simulink model "Pong3D"  (R2016b)
settings: Solver=ode45  StartTime=0.0  StopTime=10.0  FixedStep=0.001  MaxStep=updateFrequency  RelTol=1e-3  EnableMultiTasking=on
values from neighbouring files (symbols this model uses):
  Ball = struct(B_field1,B_value1,B_field2,B_value2,B_field3,B_value3,     B_field4,B_value4,B_field5,B_value5)    [PingPongStructs6DOF.m]
  Contact_Forces = struct(CF_field1,CF_value1,CF_field2,CF_value2,CF_field3,CF_value3)    [PingPongStructs6DOF.m]
  g = 9.81    [PingPongStructs6DOF.m]
  m = V(2)/V(1)    [AIPlayer.m]
  Net = struct(N_field1,N_value1)    [PingPongStructs6DOF.m]
  Robot1 = struct(R1_field1,R1_value1,R1_field2,R1_value2,R1_field3,R1_value3,     R1_field4,R1_value4, R1_field5,R1_value5,R1_field6,R1_value6,     R1_field7,R1_value7,R1_field8,R1_value8,R1_field9,R1_value9,R1_field10,R1_value10,     R1_field11,R1_value11,R1_field12,R1_value12)    [PingPongStructs6DOF.m]
  Robot2 = struct(R2_field1,R2_value1,R2_field2,R2_value2,R2_field3,R2_value3,     R2_field4, R2_value4, R2_field5,R2_value5,R2_field6,R2_value6,     R2_field7, R2_value7, R2_field8, R2_value8, R2_field9, R2_value9, R2_field10, R2_value10,     R2_field11, R2_value11, R2_field12, R2_value12)    [PingPongStructs6DOF.m]
  Table = struct(T_field1,T_value1,T_field2,T_value2)    [PingPongStructs6DOF.m]
undefined symbols (not defined in the file or in its folder): X, Y, Z
libraries: sm_lib x120, nesl_utility x55, fl_lib x48, Contact_Forces_Lib x4, Parts_Lib x3
(part 4 of 5)

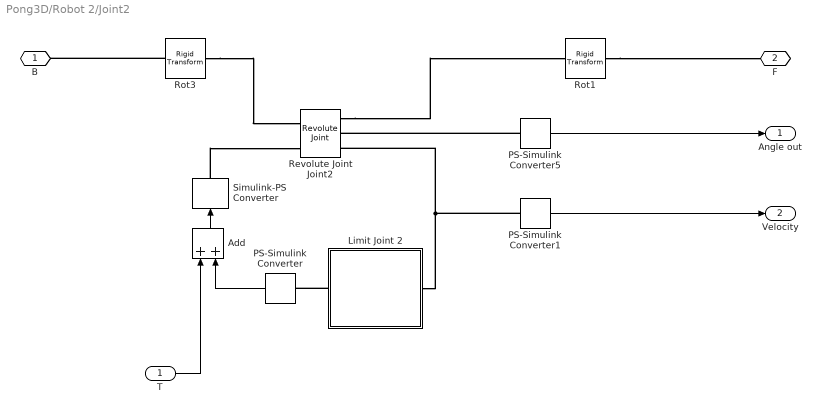
== system Pong3D/Robot 2/Joint2 ==
  T : Inport
  Add : Sum
  Limit Joint 2 : Subsystem
  PS-Simulink Converter : nesl_utility/PS-Simulink Converter  PhysicalDomain=network_engine_domain  SubClassName=ps_output  LeftPortType=input  RightPortType=output  PseudoPeriodic=off  Frequencies=[]  Unit=1  AffineConversion=off
  PS-Simulink Converter1 : nesl_utility/PS-Simulink Converter  PhysicalDomain=network_engine_domain  SubClassName=ps_output  LeftPortType=input  RightPortType=output  PseudoPeriodic=off  Frequencies=[]  Unit=1  AffineConversion=off
  PS-Simulink Converter5 : nesl_utility/PS-Simulink Converter  PhysicalDomain=network_engine_domain  SubClassName=ps_output  LeftPortType=input  RightPortType=output  PseudoPeriodic=off  Frequencies=[]  Unit=1  AffineConversion=off
  Revolute Joint Joint2 : sm_lib/Joints/Revolute Joint  SenseConstraintForce=off  SenseConstraintForceX=off  SenseConstraintForceY=off  SenseConstraintForceZ=off  SenseConstraintTorque=off  SenseConstraintTorqueX=off  SenseConstraintTorqueY=off  SenseConstraintTorqueZ=off  SenseTotalForce=off  SenseTotalForceX=off  SenseTotalForceY=off  SenseTotalForceZ=off  SenseTotalTorque=off  SenseTotalTorqueX=off  SenseTotalTorqueY=off  SenseTotalTorqueZ=off  CompositeWrenchDir=FollowerOnBase  CompositeWrenchFrame=BaseFrame  EquilibriumPosition=0  EquilibriumPositionUnits=deg  SpringStiffness=0  SpringStiffnessUnits=N*m/deg  DampingCoefficient=0  DampingCoefficientUnits=N*m/(deg/s)  TorqueActuationMode=InputTorque  MotionActuationMode=ComputedMotion  SensePosition=on  SenseVelocity=on  SenseAcceleration=off  SenseTorqueForce=off  PositionTargetSpecify=on  PositionTargetPriority=High  PositionTargetValue=Robot2.Joint.Initial_Angle(2)  PositionTargetValueUnits=deg  VelocityTargetSpecify=off  VelocityTargetPriority=High  VelocityTargetValue=0  VelocityTargetValueUnits=deg/s
  Rot1 : sm_lib/Frames and Transforms/Rigid Transform  TranslationMethod=None  TranslationStandardOffset=0  TranslationLengthUnit=m  TranslationStandardAxis=+Z  TranslationCartesianOffset=[0 0 0]  TranslationROffset=0  TranslationROffsetUnits=m  TranslationZOffset=0  TranslationZOffsetUnits=m  TranslationThetaOffset=0  TranslationThetaOffsetUnits=deg  RotationMethod=StandardAxis  RotationAngleUnits=deg  RotationStandardAxis=-X  RotationAngle=90  RotationArbitraryAxis=[0 0 1]  FollAlignAxisA=+X  BaseAlignAxisA=+Y  FollAlignAxisB=+Y  BaseAlignAxisB=+Z  RotationSequenceAxes=FollowerAxes  RotationSequence=XYX  RotationSequenceAngles=[0 0 0]  RotationSequenceAnglesUnits=deg  RotationMatrix=[1 0 0; 0 1 0; 0 0 1]
      settings: AttributesFormatString=|
      | %<RotationAngle> %<RotationAngleUnits>
      | about %<RotationStandardAxis>
  Rot3 : sm_lib/Frames and Transforms/Rigid Transform  TranslationMethod=None  TranslationStandardOffset=0  TranslationLengthUnit=m  TranslationStandardAxis=+Z  TranslationCartesianOffset=[0 0 0]  TranslationROffset=0  TranslationROffsetUnits=m  TranslationZOffset=0  TranslationZOffsetUnits=m  TranslationThetaOffset=0  TranslationThetaOffsetUnits=deg  RotationMethod=StandardAxis  RotationAngleUnits=deg  RotationStandardAxis=+X  RotationAngle=90  RotationArbitraryAxis=[0 0 1]  FollAlignAxisA=+X  BaseAlignAxisA=+Y  FollAlignAxisB=+Y  BaseAlignAxisB=+Z  RotationSequenceAxes=FollowerAxes  RotationSequence=XYX  RotationSequenceAngles=[0 0 0]  RotationSequenceAnglesUnits=deg  RotationMatrix=[1 0 0; 0 1 0; 0 0 1]
      settings: AttributesFormatString=|
      | %<RotationAngle> %<RotationAngleUnits>
      | about %<RotationStandardAxis>
  Simulink-PS Converter : nesl_utility/Simulink-PS Converter  PhysicalDomain=network_engine_domain  SubClassName=ps_input  LeftPortType=input  RightPortType=output  PseudoPeriodic=off  Frequencies=[]  NoiseDistribution=none  NoiseParameters=[]  Unit=1  AffineConversion=off  InputFiltering=off  SimscapeFilterOrder=1  InputFilterTimeConstant=0.001  UdotUserProvided=1
  B : PMIOPort  Port=1  Side=Left
  F : PMIOPort  Port=2  Side=Right
  Angle out : Outport
  Velocity : Outport  Port=2
  wires:
  Add/1 -> Simulink-PS Converter/1
  T/1 -> Add/1
  PS-Simulink Converter/1 -> Add/2
  PS-Simulink Converter5/1 -> Angle out/1
  PS-Simulink Converter1/1 -> Velocity/1
  connections:
  Rot3/LConn1 -- B/RConn1
  Limit Joint 2/RConn1 -- PS-Simulink Converter/LConn1
  Simulink-PS Converter/RConn1 -- Revolute Joint Joint2/LConn2
  Revolute Joint Joint2/RConn1 -- Rot1/LConn1
  Rot3/RConn1 -- Revolute Joint Joint2/LConn1
  Limit Joint 2/LConn1 -- PS-Simulink Converter1/LConn1 -- Revolute Joint Joint2/RConn3
  PS-Simulink Converter5/LConn1 -- Revolute Joint Joint2/RConn2
  Rot1/RConn1 -- F/RConn1

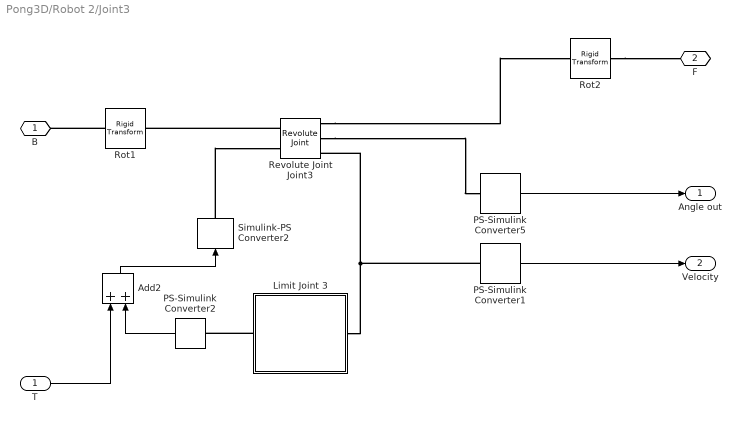
== system Pong3D/Robot 2/Joint3 ==
  T : Inport
  Add2 : Sum
  Limit Joint 3 : Subsystem
  PS-Simulink Converter1 : nesl_utility/PS-Simulink Converter  PhysicalDomain=network_engine_domain  SubClassName=ps_output  LeftPortType=input  RightPortType=output  PseudoPeriodic=off  Frequencies=[]  Unit=1  AffineConversion=off
  PS-Simulink Converter2 : nesl_utility/PS-Simulink Converter  PhysicalDomain=network_engine_domain  SubClassName=ps_output  LeftPortType=input  RightPortType=output  PseudoPeriodic=off  Frequencies=[]  Unit=1  AffineConversion=off
  PS-Simulink Converter5 : nesl_utility/PS-Simulink Converter  PhysicalDomain=network_engine_domain  SubClassName=ps_output  LeftPortType=input  RightPortType=output  PseudoPeriodic=off  Frequencies=[]  Unit=1  AffineConversion=off
  Revolute Joint Joint3 : sm_lib/Joints/Revolute Joint  SenseConstraintForce=off  SenseConstraintForceX=off  SenseConstraintForceY=off  SenseConstraintForceZ=off  SenseConstraintTorque=off  SenseConstraintTorqueX=off  SenseConstraintTorqueY=off  SenseConstraintTorqueZ=off  SenseTotalForce=off  SenseTotalForceX=off  SenseTotalForceY=off  SenseTotalForceZ=off  SenseTotalTorque=off  SenseTotalTorqueX=off  SenseTotalTorqueY=off  SenseTotalTorqueZ=off  CompositeWrenchDir=FollowerOnBase  CompositeWrenchFrame=BaseFrame  EquilibriumPosition=0  EquilibriumPositionUnits=deg  SpringStiffness=0  SpringStiffnessUnits=N*m/deg  DampingCoefficient=0  DampingCoefficientUnits=N*m/(deg/s)  TorqueActuationMode=InputTorque  MotionActuationMode=ComputedMotion  SensePosition=on  SenseVelocity=on  SenseAcceleration=off  SenseTorqueForce=off  PositionTargetSpecify=on  PositionTargetPriority=High  PositionTargetValue=Robot2.Joint.Initial_Angle(3)  PositionTargetValueUnits=deg  VelocityTargetSpecify=off  VelocityTargetPriority=High  VelocityTargetValue=0  VelocityTargetValueUnits=deg/s
  Rot1 : sm_lib/Frames and Transforms/Rigid Transform  TranslationMethod=None  TranslationStandardOffset=0  TranslationLengthUnit=m  TranslationStandardAxis=+Z  TranslationCartesianOffset=[0 0 0]  TranslationROffset=0  TranslationROffsetUnits=m  TranslationZOffset=0  TranslationZOffsetUnits=m  TranslationThetaOffset=0  TranslationThetaOffsetUnits=deg  RotationMethod=StandardAxis  RotationAngleUnits=deg  RotationStandardAxis=+X  RotationAngle=90  RotationArbitraryAxis=[0 0 1]  FollAlignAxisA=+X  BaseAlignAxisA=+Y  FollAlignAxisB=+Y  BaseAlignAxisB=+Z  RotationSequenceAxes=FollowerAxes  RotationSequence=XYX  RotationSequenceAngles=[0 0 0]  RotationSequenceAnglesUnits=deg  RotationMatrix=[1 0 0; 0 1 0; 0 0 1]
      settings: AttributesFormatString=|
      | %<RotationAngle> %<RotationAngleUnits>
      | about %<RotationStandardAxis>
  Rot2 : sm_lib/Frames and Transforms/Rigid Transform  TranslationMethod=None  TranslationStandardOffset=0  TranslationLengthUnit=m  TranslationStandardAxis=+Z  TranslationCartesianOffset=[0 0 0]  TranslationROffset=0  TranslationROffsetUnits=m  TranslationZOffset=0  TranslationZOffsetUnits=m  TranslationThetaOffset=0  TranslationThetaOffsetUnits=deg  RotationMethod=StandardAxis  RotationAngleUnits=deg  RotationStandardAxis=-X  RotationAngle=90  RotationArbitraryAxis=[0 0 1]  FollAlignAxisA=+X  BaseAlignAxisA=+Y  FollAlignAxisB=+Y  BaseAlignAxisB=+Z  RotationSequenceAxes=FollowerAxes  RotationSequence=XYX  RotationSequenceAngles=[0 0 0]  RotationSequenceAnglesUnits=deg  RotationMatrix=[1 0 0; 0 1 0; 0 0 1]
      settings: AttributesFormatString=|
      | %<RotationAngle> %<RotationAngleUnits>
      | about %<RotationStandardAxis>
  Simulink-PS Converter2 : nesl_utility/Simulink-PS Converter  PhysicalDomain=network_engine_domain  SubClassName=ps_input  LeftPortType=input  RightPortType=output  PseudoPeriodic=off  Frequencies=[]  NoiseDistribution=none  NoiseParameters=[]  Unit=1  AffineConversion=off  InputFiltering=off  SimscapeFilterOrder=1  InputFilterTimeConstant=0.001  UdotUserProvided=1
  B : PMIOPort  Port=1  Side=Left
  F : PMIOPort  Port=2  Side=Right
  Angle out : Outport
  Velocity : Outport  Port=2
  wires:
  PS-Simulink Converter2/1 -> Add2/2
  Add2/1 -> Simulink-PS Converter2/1
  T/1 -> Add2/1
  PS-Simulink Converter5/1 -> Angle out/1
  PS-Simulink Converter1/1 -> Velocity/1
  connections:
  Limit Joint 3/LConn1 -- PS-Simulink Converter1/LConn1 -- Revolute Joint Joint3/RConn3
  Revolute Joint Joint3/RConn2 -- PS-Simulink Converter5/LConn1
  Simulink-PS Converter2/RConn1 -- Revolute Joint Joint3/LConn2
  Limit Joint 3/RConn1 -- PS-Simulink Converter2/LConn1
  Rot1/LConn1 -- B/RConn1
  Revolute Joint Joint3/RConn1 -- Rot2/LConn1
  Revolute Joint Joint3/LConn1 -- Rot1/RConn1
  Rot2/RConn1 -- F/RConn1

== system Pong3D/Robot 2/Joint4 ==
  Ty : Inport
  Add3 : Sum
  Limit Joint 4 Y : Subsystem
  PS-Simulink Converter1 : nesl_utility/PS-Simulink Converter  PhysicalDomain=network_engine_domain  SubClassName=ps_output  LeftPortType=input  RightPortType=output  PseudoPeriodic=off  Frequencies=[]  Unit=1  AffineConversion=off
  PS-Simulink Converter2 : nesl_utility/PS-Simulink Converter  PhysicalDomain=network_engine_domain  SubClassName=ps_output  LeftPortType=input  RightPortType=output  PseudoPeriodic=off  Frequencies=[]  Unit=1  AffineConversion=off
  PS-Simulink Converter3 : nesl_utility/PS-Simulink Converter  PhysicalDomain=network_engine_domain  SubClassName=ps_output  LeftPortType=input  RightPortType=output  PseudoPeriodic=off  Frequencies=[]  Unit=1  AffineConversion=off
  Revolute Joint : sm_lib/Joints/Revolute Joint  SenseConstraintForce=off  SenseConstraintForceX=off  SenseConstraintForceY=off  SenseConstraintForceZ=off  SenseConstraintTorque=off  SenseConstraintTorqueX=off  SenseConstraintTorqueY=off  SenseConstraintTorqueZ=off  SenseTotalForce=off  SenseTotalForceX=off  SenseTotalForceY=off  SenseTotalForceZ=off  SenseTotalTorque=off  SenseTotalTorqueX=off  SenseTotalTorqueY=off  SenseTotalTorqueZ=off  CompositeWrenchDir=FollowerOnBase  CompositeWrenchFrame=BaseFrame  EquilibriumPosition=0  EquilibriumPositionUnits=deg  SpringStiffness=0  SpringStiffnessUnits=N*m/deg  DampingCoefficient=0  DampingCoefficientUnits=N*m/(deg/s)  TorqueActuationMode=InputTorque  MotionActuationMode=ComputedMotion  SensePosition=on  SenseVelocity=on  SenseAcceleration=off  SenseTorqueForce=off  PositionTargetSpecify=on  PositionTargetPriority=High  PositionTargetValue=Robot2.Joint.Initial_Angle(4)  PositionTargetValueUnits=deg  VelocityTargetSpecify=off  VelocityTargetPriority=High  VelocityTargetValue=0  VelocityTargetValueUnits=deg/s
  Rot1 : sm_lib/Frames and Transforms/Rigid Transform  TranslationMethod=None  TranslationStandardOffset=0  TranslationLengthUnit=m  TranslationStandardAxis=+Z  TranslationCartesianOffset=[0 0 0]  TranslationROffset=0  TranslationROffsetUnits=m  TranslationZOffset=0  TranslationZOffsetUnits=m  TranslationThetaOffset=0  TranslationThetaOffsetUnits=deg  RotationMethod=StandardAxis  RotationAngleUnits=deg  RotationStandardAxis=+X  RotationAngle=180  RotationArbitraryAxis=[0 0 1]  FollAlignAxisA=+X  BaseAlignAxisA=+Y  FollAlignAxisB=+Y  BaseAlignAxisB=+Z  RotationSequenceAxes=FollowerAxes  RotationSequence=XYX  RotationSequenceAngles=[0 0 0]  RotationSequenceAnglesUnits=deg  RotationMatrix=[1 0 0; 0 1 0; 0 0 1]
      settings: AttributesFormatString=|
      | %<RotationAngle> %<RotationAngleUnits>
      | about %<RotationStandardAxis>
  Rot2 : sm_lib/Frames and Transforms/Rigid Transform  TranslationMethod=None  TranslationStandardOffset=0  TranslationLengthUnit=m  TranslationStandardAxis=+Z  TranslationCartesianOffset=[0 0 0]  TranslationROffset=0  TranslationROffsetUnits=m  TranslationZOffset=0  TranslationZOffsetUnits=m  TranslationThetaOffset=0  TranslationThetaOffsetUnits=deg  RotationMethod=StandardAxis  RotationAngleUnits=deg  RotationStandardAxis=-X  RotationAngle=180  RotationArbitraryAxis=[0 0 1]  FollAlignAxisA=+X  BaseAlignAxisA=+Y  FollAlignAxisB=+Y  BaseAlignAxisB=+Z  RotationSequenceAxes=FollowerAxes  RotationSequence=XYX  RotationSequenceAngles=[0 0 0]  RotationSequenceAnglesUnits=deg  RotationMatrix=[1 0 0; 0 1 0; 0 0 1]
      settings: AttributesFormatString=|
      | %<RotationAngle> %<RotationAngleUnits>
      | about %<RotationStandardAxis>
  Simulink-PS Converter3 : nesl_utility/Simulink-PS Converter  PhysicalDomain=network_engine_domain  SubClassName=ps_input  LeftPortType=input  RightPortType=output  PseudoPeriodic=off  Frequencies=[]  NoiseDistribution=none  NoiseParameters=[]  Unit=1  AffineConversion=off  InputFiltering=off  SimscapeFilterOrder=1  InputFilterTimeConstant=0.001  UdotUserProvided=1
  B : PMIOPort  Port=1  Side=Left
  F : PMIOPort  Port=2  Side=Right
  Angle Y out : Outport
  Velocity : Outport  Port=2
  wires:
  Add3/1 -> Simulink-PS Converter3/1
  PS-Simulink Converter3/1 -> Add3/2
  PS-Simulink Converter1/1 -> Angle Y out/1
  Ty/1 -> Add3/1
  PS-Simulink Converter2/1 -> Velocity/1
  connections:
  Rot2/RConn1 -- F/RConn1
  Limit Joint 4 Y/RConn1 -- PS-Simulink Converter3/LConn1
  Rot1/RConn1 -- Revolute Joint/LConn1
  PS-Simulink Converter1/LConn1 -- Revolute Joint/RConn2
  Limit Joint 4 Y/LConn1 -- Revolute Joint/RConn3 -- PS-Simulink Converter2/LConn1
  Simulink-PS Converter3/RConn1 -- Revolute Joint/LConn2
  B/RConn1 -- Rot1/LConn1
  Revolute Joint/RConn1 -- Rot2/LConn1

== system Pong3D/Robot 2/Joint5 ==
  Ty : Inport
  Add3 : Sum
  Limit Joint 4 Y : Subsystem
  PS-Simulink Converter1 : nesl_utility/PS-Simulink Converter  PhysicalDomain=network_engine_domain  SubClassName=ps_output  LeftPortType=input  RightPortType=output  PseudoPeriodic=off  Frequencies=[]  Unit=1  AffineConversion=off
  PS-Simulink Converter2 : nesl_utility/PS-Simulink Converter  PhysicalDomain=network_engine_domain  SubClassName=ps_output  LeftPortType=input  RightPortType=output  PseudoPeriodic=off  Frequencies=[]  Unit=1  AffineConversion=off
  PS-Simulink Converter3 : nesl_utility/PS-Simulink Converter  PhysicalDomain=network_engine_domain  SubClassName=ps_output  LeftPortType=input  RightPortType=output  PseudoPeriodic=off  Frequencies=[]  Unit=1  AffineConversion=off
  Revolute Joint : sm_lib/Joints/Revolute Joint  SenseConstraintForce=off  SenseConstraintForceX=off  SenseConstraintForceY=off  SenseConstraintForceZ=off  SenseConstraintTorque=off  SenseConstraintTorqueX=off  SenseConstraintTorqueY=off  SenseConstraintTorqueZ=off  SenseTotalForce=off  SenseTotalForceX=off  SenseTotalForceY=off  SenseTotalForceZ=off  SenseTotalTorque=off  SenseTotalTorqueX=off  SenseTotalTorqueY=off  SenseTotalTorqueZ=off  CompositeWrenchDir=FollowerOnBase  CompositeWrenchFrame=BaseFrame  EquilibriumPosition=0  EquilibriumPositionUnits=deg  SpringStiffness=0  SpringStiffnessUnits=N*m/deg  DampingCoefficient=0  DampingCoefficientUnits=N*m/(deg/s)  TorqueActuationMode=InputTorque  MotionActuationMode=ComputedMotion  SensePosition=on  SenseVelocity=on  SenseAcceleration=off  SenseTorqueForce=off  PositionTargetSpecify=on  PositionTargetPriority=High  PositionTargetValue=Robot2.Joint.Initial_Angle(5)  PositionTargetValueUnits=deg  VelocityTargetSpecify=off  VelocityTargetPriority=High  VelocityTargetValue=0  VelocityTargetValueUnits=deg/s
  Rot1 : sm_lib/Frames and Transforms/Rigid Transform  TranslationMethod=None  TranslationStandardOffset=0  TranslationLengthUnit=m  TranslationStandardAxis=+Z  TranslationCartesianOffset=[0 0 0]  TranslationROffset=0  TranslationROffsetUnits=m  TranslationZOffset=0  TranslationZOffsetUnits=m  TranslationThetaOffset=0  TranslationThetaOffsetUnits=deg  RotationMethod=StandardAxis  RotationAngleUnits=deg  RotationStandardAxis=-X  RotationAngle=90  RotationArbitraryAxis=[0 0 1]  FollAlignAxisA=+X  BaseAlignAxisA=+Y  FollAlignAxisB=+Y  BaseAlignAxisB=+Z  RotationSequenceAxes=FollowerAxes  RotationSequence=XYX  RotationSequenceAngles=[0 0 0]  RotationSequenceAnglesUnits=deg  RotationMatrix=[1 0 0; 0 1 0; 0 0 1]
      settings: AttributesFormatString=|
      | %<RotationAngle> %<RotationAngleUnits>
      | about %<RotationStandardAxis>
  Rot3 : sm_lib/Frames and Transforms/Rigid Transform  TranslationMethod=None  TranslationStandardOffset=0  TranslationLengthUnit=m  TranslationStandardAxis=+Z  TranslationCartesianOffset=[0 0 0]  TranslationROffset=0  TranslationROffsetUnits=m  TranslationZOffset=0  TranslationZOffsetUnits=m  TranslationThetaOffset=0  TranslationThetaOffsetUnits=deg  RotationMethod=StandardAxis  RotationAngleUnits=deg  RotationStandardAxis=+X  RotationAngle=90  RotationArbitraryAxis=[0 0 1]  FollAlignAxisA=+X  BaseAlignAxisA=+Y  FollAlignAxisB=+Y  BaseAlignAxisB=+Z  RotationSequenceAxes=FollowerAxes  RotationSequence=XYX  RotationSequenceAngles=[0 0 0]  RotationSequenceAnglesUnits=deg  RotationMatrix=[1 0 0; 0 1 0; 0 0 1]
      settings: AttributesFormatString=|
      | %<RotationAngle> %<RotationAngleUnits>
      | about %<RotationStandardAxis>
  Simulink-PS Converter3 : nesl_utility/Simulink-PS Converter  PhysicalDomain=network_engine_domain  SubClassName=ps_input  LeftPortType=input  RightPortType=output  PseudoPeriodic=off  Frequencies=[]  NoiseDistribution=none  NoiseParameters=[]  Unit=1  AffineConversion=off  InputFiltering=off  SimscapeFilterOrder=1  InputFilterTimeConstant=0.001  UdotUserProvided=1
  B : PMIOPort  Port=1  Side=Left
  F : PMIOPort  Port=2  Side=Right
  Angle Y out : Outport
  Velocity : Outport  Port=2
  wires:
  Ty/1 -> Add3/1
  PS-Simulink Converter1/1 -> Angle Y out/1
  PS-Simulink Converter3/1 -> Add3/2
  Add3/1 -> Simulink-PS Converter3/1
  PS-Simulink Converter2/1 -> Velocity/1
  connections:
  Simulink-PS Converter3/RConn1 -- Revolute Joint/LConn2
  Limit Joint 4 Y/LConn1 -- PS-Simulink Converter2/LConn1 -- Revolute Joint/RConn3
  PS-Simulink Converter1/LConn1 -- Revolute Joint/RConn2
  Limit Joint 4 Y/RConn1 -- PS-Simulink Converter3/LConn1
  Revolute Joint/RConn1 -- Rot1/LConn1
  B/RConn1 -- Rot3/LConn1
  Rot3/RConn1 -- Revolute Joint/LConn1
  Rot1/RConn1 -- F/RConn1

== system Pong3D/Robot 2/Joint6 ==
  Ty : Inport
  Add3 : Sum
  Limit Joint 4 Y : Subsystem
  PS-Simulink Converter1 : nesl_utility/PS-Simulink Converter  PhysicalDomain=network_engine_domain  SubClassName=ps_output  LeftPortType=input  RightPortType=output  PseudoPeriodic=off  Frequencies=[]  Unit=1  AffineConversion=off
  PS-Simulink Converter2 : nesl_utility/PS-Simulink Converter  PhysicalDomain=network_engine_domain  SubClassName=ps_output  LeftPortType=input  RightPortType=output  PseudoPeriodic=off  Frequencies=[]  Unit=1  AffineConversion=off
  PS-Simulink Converter3 : nesl_utility/PS-Simulink Converter  PhysicalDomain=network_engine_domain  SubClassName=ps_output  LeftPortType=input  RightPortType=output  PseudoPeriodic=off  Frequencies=[]  Unit=1  AffineConversion=off
  Revolute Joint : sm_lib/Joints/Revolute Joint  SenseConstraintForce=off  SenseConstraintForceX=off  SenseConstraintForceY=off  SenseConstraintForceZ=off  SenseConstraintTorque=off  SenseConstraintTorqueX=off  SenseConstraintTorqueY=off  SenseConstraintTorqueZ=off  SenseTotalForce=off  SenseTotalForceX=off  SenseTotalForceY=off  SenseTotalForceZ=off  SenseTotalTorque=off  SenseTotalTorqueX=off  SenseTotalTorqueY=off  SenseTotalTorqueZ=off  CompositeWrenchDir=FollowerOnBase  CompositeWrenchFrame=BaseFrame  EquilibriumPosition=0  EquilibriumPositionUnits=deg  SpringStiffness=0  SpringStiffnessUnits=N*m/deg  DampingCoefficient=0  DampingCoefficientUnits=N*m/(deg/s)  TorqueActuationMode=InputTorque  MotionActuationMode=ComputedMotion  SensePosition=on  SenseVelocity=on  SenseAcceleration=off  SenseTorqueForce=off  PositionTargetSpecify=on  PositionTargetPriority=High  PositionTargetValue=Robot2.Joint.Initial_Angle(6)  PositionTargetValueUnits=deg  VelocityTargetSpecify=off  VelocityTargetPriority=High  VelocityTargetValue=0  VelocityTargetValueUnits=deg/s
  Rot1 : sm_lib/Frames and Transforms/Rigid Transform  TranslationMethod=None  TranslationStandardOffset=0  TranslationLengthUnit=m  TranslationStandardAxis=+Z  TranslationCartesianOffset=[0 0 0]  TranslationROffset=0  TranslationROffsetUnits=m  TranslationZOffset=0  TranslationZOffsetUnits=m  TranslationThetaOffset=0  TranslationThetaOffsetUnits=deg  RotationMethod=StandardAxis  RotationAngleUnits=deg  RotationStandardAxis=+X  RotationAngle=180  RotationArbitraryAxis=[0 0 1]  FollAlignAxisA=+X  BaseAlignAxisA=+Y  FollAlignAxisB=+Y  BaseAlignAxisB=+Z  RotationSequenceAxes=FollowerAxes  RotationSequence=XYX  RotationSequenceAngles=[0 0 0]  RotationSequenceAnglesUnits=deg  RotationMatrix=[1 0 0; 0 1 0; 0 0 1]
      settings: AttributesFormatString=|
      | %<RotationAngle> %<RotationAngleUnits>
      | about %<RotationStandardAxis>
  Rot2 : sm_lib/Frames and Transforms/Rigid Transform  TranslationMethod=None  TranslationStandardOffset=0  TranslationLengthUnit=m  TranslationStandardAxis=+Z  TranslationCartesianOffset=[0 0 0]  TranslationROffset=0  TranslationROffsetUnits=m  TranslationZOffset=0  TranslationZOffsetUnits=m  TranslationThetaOffset=0  TranslationThetaOffsetUnits=deg  RotationMethod=StandardAxis  RotationAngleUnits=deg  RotationStandardAxis=-X  RotationAngle=180  RotationArbitraryAxis=[0 0 1]  FollAlignAxisA=+X  BaseAlignAxisA=+Y  FollAlignAxisB=+Y  BaseAlignAxisB=+Z  RotationSequenceAxes=FollowerAxes  RotationSequence=XYX  RotationSequenceAngles=[0 0 0]  RotationSequenceAnglesUnits=deg  RotationMatrix=[1 0 0; 0 1 0; 0 0 1]
      settings: AttributesFormatString=|
      | %<RotationAngle> %<RotationAngleUnits>
      | about %<RotationStandardAxis>
  Simulink-PS Converter3 : nesl_utility/Simulink-PS Converter  PhysicalDomain=network_engine_domain  SubClassName=ps_input  LeftPortType=input  RightPortType=output  PseudoPeriodic=off  Frequencies=[]  NoiseDistribution=none  NoiseParameters=[]  Unit=1  AffineConversion=off  InputFiltering=off  SimscapeFilterOrder=1  InputFilterTimeConstant=0.001  UdotUserProvided=1
  B : PMIOPort  Port=1  Side=Left
  F : PMIOPort  Port=2  Side=Right
  Angle Y out : Outport
  Velocity : Outport  Port=2
  wires:
  Ty/1 -> Add3/1
  PS-Simulink Converter1/1 -> Angle Y out/1
  PS-Simulink Converter3/1 -> Add3/2
  Add3/1 -> Simulink-PS Converter3/1
  PS-Simulink Converter2/1 -> Velocity/1
  connections:
  Simulink-PS Converter3/RConn1 -- Revolute Joint/LConn2
  Limit Joint 4 Y/LConn1 -- PS-Simulink Converter2/LConn1 -- Revolute Joint/RConn3
  PS-Simulink Converter1/LConn1 -- Revolute Joint/RConn2
  Limit Joint 4 Y/RConn1 -- PS-Simulink Converter3/LConn1
  B/RConn1 -- Rot1/LConn1
  Rot2/RConn1 -- F/RConn1
  Rot1/RConn1 -- Revolute Joint/LConn1
  Revolute Joint/RConn1 -- Rot2/LConn1

== system Pong3D/Robot 2/Paddle1 ==
  Paddle1 : Parts_Lib/Cylinder  Tag=CustomStyle  cyl_radius=Robot2.Paddle(1)  cyl_length=Robot2.Paddle(2)  cyl_density=Robot2.Paddle(3)  cyl_color=blue  cyl_opacity=1  mark_radius=[0.75 0.5]  mark_angle=60  mark_color=purple  mark_opacity=1
  Rot1 : sm_lib/Frames and Transforms/Rigid Transform  TranslationMethod=None  TranslationStandardOffset=0  TranslationLengthUnit=m  TranslationStandardAxis=+Z  TranslationCartesianOffset=[0 0 0]  TranslationROffset=0  TranslationROffsetUnits=m  TranslationZOffset=0  TranslationZOffsetUnits=m  TranslationThetaOffset=0  TranslationThetaOffsetUnits=deg  RotationMethod=StandardAxis  RotationAngleUnits=deg  RotationStandardAxis=+Y  RotationAngle=180  RotationArbitraryAxis=[0 0 1]  FollAlignAxisA=+X  BaseAlignAxisA=+Y  FollAlignAxisB=+Y  BaseAlignAxisB=+Z  RotationSequenceAxes=FollowerAxes  RotationSequence=XYX  RotationSequenceAngles=[0 0 0]  RotationSequenceAnglesUnits=deg  RotationMatrix=[1 0 0; 0 1 0; 0 0 1]
      settings: AttributesFormatString=|
      | %<RotationAngle> %<RotationAngleUnits>
      | about %<RotationStandardAxis>
  Rot2 : sm_lib/Frames and Transforms/Rigid Transform  TranslationMethod=None  TranslationStandardOffset=0  TranslationLengthUnit=m  TranslationStandardAxis=+Z  TranslationCartesianOffset=[0 0 0]  TranslationROffset=0  TranslationROffsetUnits=m  TranslationZOffset=0  TranslationZOffsetUnits=m  TranslationThetaOffset=0  TranslationThetaOffsetUnits=deg  RotationMethod=StandardAxis  RotationAngleUnits=deg  RotationStandardAxis=-Y  RotationAngle=90  RotationArbitraryAxis=[0 0 1]  FollAlignAxisA=+X  BaseAlignAxisA=+Y  FollAlignAxisB=+Y  BaseAlignAxisB=+Z  RotationSequenceAxes=FollowerAxes  RotationSequence=XYX  RotationSequenceAngles=[0 0 0]  RotationSequenceAnglesUnits=deg  RotationMatrix=[1 0 0; 0 1 0; 0 0 1]
      settings: AttributesFormatString=|
      | %<RotationAngle> %<RotationAngleUnits>
      | about %<RotationStandardAxis>
  Trans1 : sm_lib/Frames and Transforms/Rigid Transform  TranslationMethod=StandardAxis  TranslationStandardOffset=Robot2.Paddle(1)  TranslationLengthUnit=m  TranslationStandardAxis=+Z  TranslationCartesianOffset=[0 0 0]  TranslationROffset=0  TranslationROffsetUnits=m  TranslationZOffset=0  TranslationZOffsetUnits=m  TranslationThetaOffset=0  TranslationThetaOffsetUnits=deg  RotationMethod=None  RotationAngleUnits=deg  RotationStandardAxis=+Z  RotationAngle=0.0  RotationArbitraryAxis=[0 0 1]  FollAlignAxisA=+X  BaseAlignAxisA=+Y  FollAlignAxisB=+Y  BaseAlignAxisB=+Z  RotationSequenceAxes=FollowerAxes  RotationSequence=XYX  RotationSequenceAngles=[0 0 0]  RotationSequenceAnglesUnits=deg  RotationMatrix=[1 0 0; 0 1 0; 0 0 1]
      settings: AttributesFormatString=|
      | %<TranslationStandardOffset> %<TranslationLengthUnit>
      | in %<TranslationStandardAxis>
  B : PMIOPort  Port=1  Side=Left
  connections:
  Rot1/LConn1 -- B/RConn1
  Trans1/RConn1 -- Rot2/LConn1
  Rot1/RConn1 -- Trans1/LConn1
  Rot2/RConn1 -- Paddle1/LConn1

== system Pong3D/Subsystem3/Subsystem1 ==
  Fdbk Angle : Inport
  Debk Velocity : Inport  Port=2
  Angle : Inport  Port=3
  Velocity : Inport  Port=4
  Torque : Inport  Port=5
  Add : Sum  Inputs=-+
  Add1 : Sum  Inputs=-+
  Add2 : Sum
  Add3 : Sum
  Kd : Gain  Gain=300
  Kp : Gain  Gain=10000
  Torq : Outport
  wires:
  Fdbk Angle/1 -> Add/1
  Add/1 -> Kp/1
  Debk Velocity/1 -> Add1/1
  Angle/1 -> Add/2
  Velocity/1 -> Add1/2
  Torque/1 -> Add3/2
  Kd/1 -> Add2/2
  Add3/1 -> Torq/1
  Kp/1 -> Add2/1
  Add2/1 -> Add3/1
  Add1/1 -> Kd/1

== system Pong3D/Subsystem3/Subsystem2 ==
  Fdbk Angle : Inport
  Debk Velocity : Inport  Port=2
  Angle : Inport  Port=3
  Velocity : Inport  Port=4
  Torque : Inport  Port=5
  Add : Sum  Inputs=-+
  Add1 : Sum  Inputs=-+
  Add2 : Sum
  Add3 : Sum
  Kd : Gain  Gain=500
  Kp : Gain  Gain=10000
  Torq : Outport
  wires:
  Add1/1 -> Kd/1
  Add2/1 -> Add3/1
  Kp/1 -> Add2/1
  Add3/1 -> Torq/1
  Kd/1 -> Add2/2
  Torque/1 -> Add3/2
  Velocity/1 -> Add1/2
  Angle/1 -> Add/2
  Debk Velocity/1 -> Add1/1
  Add/1 -> Kp/1
  Fdbk Angle/1 -> Add/1

== system Pong3D/Subsystem3/Subsystem3 ==
  Fdbk Angle : Inport
  Debk Velocity : Inport  Port=2
  Angle : Inport  Port=3
  Velocity : Inport  Port=4
  Torque : Inport  Port=5
  Add : Sum  Inputs=-+
  Add1 : Sum  Inputs=-+
  Add2 : Sum
  Add3 : Sum
  Kd : Gain  Gain=30
  Kp : Gain  Gain=800
  Torq : Outport
  wires:
  Fdbk Angle/1 -> Add/1
  Add/1 -> Kp/1
  Debk Velocity/1 -> Add1/1
  Angle/1 -> Add/2
  Velocity/1 -> Add1/2
  Torque/1 -> Add3/2
  Kd/1 -> Add2/2
  Add3/1 -> Torq/1
  Kp/1 -> Add2/1
  Add2/1 -> Add3/1
  Add1/1 -> Kd/1

== system Pong3D/Subsystem3/Subsystem4 ==
  Fdbk Angle : Inport
  Debk Velocity : Inport  Port=2
  Angle : Inport  Port=3
  Velocity : Inport  Port=4
  Torque : Inport  Port=5
  Add : Sum  Inputs=-+
  Add1 : Sum  Inputs=-+
  Add2 : Sum
  Add3 : Sum
  Kd : Gain
  Kp : Gain  Gain=100
  Torq : Outport
  wires:
  Add1/1 -> Kd/1
  Add2/1 -> Add3/1
  Kp/1 -> Add2/1
  Add3/1 -> Torq/1
  Kd/1 -> Add2/2
  Torque/1 -> Add3/2
  Velocity/1 -> Add1/2
  Angle/1 -> Add/2
  Debk Velocity/1 -> Add1/1
  Add/1 -> Kp/1
  Fdbk Angle/1 -> Add/1

== system Pong3D/Subsystem3/Subsystem5 ==
  Fdbk Angle : Inport
  Debk Velocity : Inport  Port=2
  Angle : Inport  Port=3
  Velocity : Inport  Port=4
  Torque : Inport  Port=5
  Add : Sum  Inputs=-+
  Add1 : Sum  Inputs=-+
  Add2 : Sum
  Add3 : Sum
  Kd : Gain
  Kp : Gain  Gain=75
  Torq : Outport
  wires:
  Fdbk Angle/1 -> Add/1
  Add/1 -> Kp/1
  Debk Velocity/1 -> Add1/1
  Angle/1 -> Add/2
  Velocity/1 -> Add1/2
  Torque/1 -> Add3/2
  Kd/1 -> Add2/2
  Add3/1 -> Torq/1
  Kp/1 -> Add2/1
  Add2/1 -> Add3/1
  Add1/1 -> Kd/1

== system Pong3D/Subsystem3/Subsystem6 ==
  Fdbk Angle : Inport
  Debk Velocity : Inport  Port=2
  Angle : Inport  Port=3
  Velocity : Inport  Port=4
  Torque : Inport  Port=5
  Add : Sum  Inputs=-+
  Add1 : Sum  Inputs=-+
  Add2 : Sum
  Add3 : Sum
  Kd : Gain
  Kp : Gain  Gain=50
  Torq : Outport
  wires:
  Add1/1 -> Kd/1
  Add2/1 -> Add3/1
  Kp/1 -> Add2/1
  Add3/1 -> Torq/1
  Kd/1 -> Add2/2
  Torque/1 -> Add3/2
  Velocity/1 -> Add1/2
  Angle/1 -> Add/2
  Debk Velocity/1 -> Add1/1
  Add/1 -> Kp/1
  Fdbk Angle/1 -> Add/1

== system Pong3D/Subsystem4/Subsystem1 ==
  Fdbk Angle : Inport
  Debk Velocity : Inport  Port=2
  Angle : Inport  Port=3
  Velocity : Inport  Port=4
  Torque : Inport  Port=5
  Add : Sum  Inputs=-+
  Add1 : Sum  Inputs=-+
  Add2 : Sum
  Add3 : Sum
  Kd : Gain  Gain=300
  Kp : Gain  Gain=10000
  Torq : Outport
  wires:
  Add1/1 -> Kd/1
  Add2/1 -> Add3/1
  Kp/1 -> Add2/1
  Add3/1 -> Torq/1
  Kd/1 -> Add2/2
  Torque/1 -> Add3/2
  Velocity/1 -> Add1/2
  Angle/1 -> Add/2
  Debk Velocity/1 -> Add1/1
  Add/1 -> Kp/1
  Fdbk Angle/1 -> Add/1

== system Pong3D/Subsystem4/Subsystem2 ==
  Fdbk Angle : Inport
  Debk Velocity : Inport  Port=2
  Angle : Inport  Port=3
  Velocity : Inport  Port=4
  Torque : Inport  Port=5
  Add : Sum  Inputs=-+
  Add1 : Sum  Inputs=-+
  Add2 : Sum
  Add3 : Sum
  Kd : Gain  Gain=500
  Kp : Gain  Gain=10000
  Torq : Outport
  wires:
  Fdbk Angle/1 -> Add/1
  Add/1 -> Kp/1
  Debk Velocity/1 -> Add1/1
  Angle/1 -> Add/2
  Velocity/1 -> Add1/2
  Torque/1 -> Add3/2
  Kd/1 -> Add2/2
  Add3/1 -> Torq/1
  Kp/1 -> Add2/1
  Add2/1 -> Add3/1
  Add1/1 -> Kd/1

== system Pong3D/Subsystem4/Subsystem3 ==
  Fdbk Angle : Inport
  Debk Velocity : Inport  Port=2
  Angle : Inport  Port=3
  Velocity : Inport  Port=4
  Torque : Inport  Port=5
  Add : Sum  Inputs=-+
  Add1 : Sum  Inputs=-+
  Add2 : Sum
  Add3 : Sum
  Kd : Gain  Gain=30
  Kp : Gain  Gain=800
  Torq : Outport
  wires:
  Add1/1 -> Kd/1
  Add2/1 -> Add3/1
  Kp/1 -> Add2/1
  Add3/1 -> Torq/1
  Kd/1 -> Add2/2
  Torque/1 -> Add3/2
  Velocity/1 -> Add1/2
  Angle/1 -> Add/2
  Debk Velocity/1 -> Add1/1
  Add/1 -> Kp/1
  Fdbk Angle/1 -> Add/1

== system Pong3D/Subsystem4/Subsystem4 ==
  Fdbk Angle : Inport
  Debk Velocity : Inport  Port=2
  Angle : Inport  Port=3
  Velocity : Inport  Port=4
  Torque : Inport  Port=5
  Add : Sum  Inputs=-+
  Add1 : Sum  Inputs=-+
  Add2 : Sum
  Add3 : Sum
  Kd : Gain
  Kp : Gain  Gain=100
  Torq : Outport
  wires:
  Fdbk Angle/1 -> Add/1
  Add/1 -> Kp/1
  Debk Velocity/1 -> Add1/1
  Angle/1 -> Add/2
  Velocity/1 -> Add1/2
  Torque/1 -> Add3/2
  Kd/1 -> Add2/2
  Add3/1 -> Torq/1
  Kp/1 -> Add2/1
  Add2/1 -> Add3/1
  Add1/1 -> Kd/1

== system Pong3D/Subsystem4/Subsystem5 ==
  Fdbk Angle : Inport
  Debk Velocity : Inport  Port=2
  Angle : Inport  Port=3
  Velocity : Inport  Port=4
  Torque : Inport  Port=5
  Add : Sum  Inputs=-+
  Add1 : Sum  Inputs=-+
  Add2 : Sum
  Add3 : Sum
  Kd : Gain
  Kp : Gain  Gain=75
  Torq : Outport
  wires:
  Add1/1 -> Kd/1
  Add2/1 -> Add3/1
  Kp/1 -> Add2/1
  Add3/1 -> Torq/1
  Kd/1 -> Add2/2
  Torque/1 -> Add3/2
  Velocity/1 -> Add1/2
  Angle/1 -> Add/2
  Debk Velocity/1 -> Add1/1
  Add/1 -> Kp/1
  Fdbk Angle/1 -> Add/1

== system Pong3D/Subsystem4/Subsystem6 ==
  Fdbk Angle : Inport
  Debk Velocity : Inport  Port=2
  Angle : Inport  Port=3
  Velocity : Inport  Port=4
  Torque : Inport  Port=5
  Add : Sum  Inputs=-+
  Add1 : Sum  Inputs=-+
  Add2 : Sum
  Add3 : Sum
  Kd : Gain
  Kp : Gain  Gain=50
  Torq : Outport
  wires:
  Fdbk Angle/1 -> Add/1
  Add/1 -> Kp/1
  Debk Velocity/1 -> Add1/1
  Angle/1 -> Add/2
  Velocity/1 -> Add1/2
  Torque/1 -> Add3/2
  Kd/1 -> Add2/2
  Add3/1 -> Torq/1
  Kp/1 -> Add2/1
  Add2/1 -> Add3/1
  Add1/1 -> Kd/1

== system Pong3D/Robot 1/Joint1/Limit Joint 1 ==
  Ideal Angular Velocity Source : fl_lib/Mechanical/Mechanical Sources/Ideal Angular Velocity Source
  Ideal Torque Sensor : fl_lib/Mechanical/Mechanical Sensors/Ideal Torque Sensor
  Mechanical Rotational Reference : fl_lib/Mechanical/Rotational Elements/Mechanical Rotational Reference
  Rotational Hard Stop1 : fl_lib/Mechanical/Rotational Elements/Rotational Hard Stop  upper_bnd=Robot1.Joint.Upper_Bound(1) - Robot1.Joint.Initial_Angle(1) deg  lower_bnd=Robot1.Joint.Lower_Bound(1) - Robot1.Joint.Initial_Angle(1) deg  stiff_up=Robot1.Joint.Contact_Stiffness(1) N*m/rad  stiff_low=Robot1.Joint.Contact_Stiffness(1) N*m/rad  D_up=Robot1.Joint.Contact_Damping(1) N*m/(rad/s)  D_low=Robot1.Joint.Contact_Damping(1) N*m/(rad/s)  w_specify=off  w_priority=High  w=0 rad/s  t_specify=off  t_priority=High  t=0 N*m  phi_specify=off  phi_priority=High  phi=0 rad
  T : PMIOPort  Port=1  Side=Right
  W : PMIOPort  Port=2  Side=Left
  connections:
  W/RConn1 -- Ideal Angular Velocity Source/RConn1
  Ideal Angular Velocity Source/LConn1 -- Mechanical Rotational Reference/LConn1 -- Rotational Hard Stop1/LConn1
  Rotational Hard Stop1/RConn1 -- Ideal Torque Sensor/RConn1
  Ideal Torque Sensor/RConn2 -- T/RConn1
  Ideal Torque Sensor/LConn1 -- Ideal Angular Velocity Source/RConn2

== system Pong3D/Robot 1/Joint2/Limit Joint 2 ==
  Ideal Angular Velocity Source : fl_lib/Mechanical/Mechanical Sources/Ideal Angular Velocity Source
  Ideal Torque Sensor : fl_lib/Mechanical/Mechanical Sensors/Ideal Torque Sensor
  Mechanical Rotational Reference : fl_lib/Mechanical/Rotational Elements/Mechanical Rotational Reference
  Rotational Hard Stop1 : fl_lib/Mechanical/Rotational Elements/Rotational Hard Stop  upper_bnd=Robot1.Joint.Upper_Bound(2) - Robot1.Joint.Initial_Angle(2) deg  lower_bnd=Robot1.Joint.Lower_Bound(2) - Robot1.Joint.Initial_Angle(2) deg  stiff_up=Robot1.Joint.Contact_Stiffness(2) N*m/rad  stiff_low=Robot1.Joint.Contact_Stiffness(2) N*m/rad  D_up=Robot1.Joint.Contact_Damping(2) N*m/(rad/s)  D_low=Robot1.Joint.Contact_Damping(2) N*m/(rad/s)  w_specify=off  w_priority=High  w=0 rad/s  t_specify=off  t_priority=High  t=0 N*m  phi_specify=off  phi_priority=High  phi=0 rad
  T : PMIOPort  Port=1  Side=Right
  W : PMIOPort  Port=2  Side=Left
  connections:
  Ideal Torque Sensor/LConn1 -- Ideal Angular Velocity Source/RConn2
  Ideal Torque Sensor/RConn2 -- T/RConn1
  Rotational Hard Stop1/RConn1 -- Ideal Torque Sensor/RConn1
  Rotational Hard Stop1/LConn1 -- Mechanical Rotational Reference/LConn1 -- Ideal Angular Velocity Source/LConn1
  W/RConn1 -- Ideal Angular Velocity Source/RConn1

== system Pong3D/Robot 1/Joint3/Limit Joint 3 ==
  Ideal Angular Velocity Source : fl_lib/Mechanical/Mechanical Sources/Ideal Angular Velocity Source
  Ideal Torque Sensor : fl_lib/Mechanical/Mechanical Sensors/Ideal Torque Sensor
  Mechanical Rotational Reference : fl_lib/Mechanical/Rotational Elements/Mechanical Rotational Reference
  Rotational Hard Stop1 : fl_lib/Mechanical/Rotational Elements/Rotational Hard Stop  upper_bnd=Robot1.Joint.Upper_Bound(3) - Robot1.Joint.Initial_Angle(3) deg  lower_bnd=Robot1.Joint.Lower_Bound(3) - Robot1.Joint.Initial_Angle(3) deg  stiff_up=Robot1.Joint.Contact_Stiffness(3) N*m/rad  stiff_low=Robot1.Joint.Contact_Stiffness(3) N*m/rad  D_up=Robot1.Joint.Contact_Damping(3) N*m/(rad/s)  D_low=Robot1.Joint.Contact_Damping(3) N*m/(rad/s)  w_specify=off  w_priority=High  w=0 rad/s  t_specify=off  t_priority=High  t=0 N*m  phi_specify=off  phi_priority=High  phi=0 rad
  T : PMIOPort  Port=1  Side=Right
  W : PMIOPort  Port=2  Side=Left
  connections:
  W/RConn1 -- Ideal Angular Velocity Source/RConn1
  Ideal Angular Velocity Source/LConn1 -- Mechanical Rotational Reference/LConn1 -- Rotational Hard Stop1/LConn1
  Rotational Hard Stop1/RConn1 -- Ideal Torque Sensor/RConn1
  Ideal Torque Sensor/RConn2 -- T/RConn1
  Ideal Torque Sensor/LConn1 -- Ideal Angular Velocity Source/RConn2

== system Pong3D/Robot 1/Joint4/Limit Joint 4 ==
  Ideal Angular Velocity Source : fl_lib/Mechanical/Mechanical Sources/Ideal Angular Velocity Source
  Ideal Torque Sensor : fl_lib/Mechanical/Mechanical Sensors/Ideal Torque Sensor
  Mechanical Rotational Reference : fl_lib/Mechanical/Rotational Elements/Mechanical Rotational Reference
  Rotational Hard Stop1 : fl_lib/Mechanical/Rotational Elements/Rotational Hard Stop  upper_bnd=Robot1.Joint.Upper_Bound(4) - Robot1.Joint.Initial_Angle(4) deg  lower_bnd=Robot1.Joint.Lower_Bound(4) - Robot1.Joint.Initial_Angle(4) deg  stiff_up=Robot1.Joint.Contact_Stiffness(4) N*m/rad  stiff_low=Robot1.Joint.Contact_Stiffness(4) N*m/rad  D_up=Robot1.Joint.Contact_Damping(4) N*m/(rad/s)  D_low=Robot1.Joint.Contact_Damping(4) N*m/(rad/s)  w_specify=off  w_priority=High  w=0 rad/s  t_specify=off  t_priority=High  t=0 N*m  phi_specify=off  phi_priority=High  phi=0 rad
  T : PMIOPort  Port=1  Side=Right
  W : PMIOPort  Port=2  Side=Left
  connections:
  W/RConn1 -- Ideal Angular Velocity Source/RConn1
  Ideal Angular Velocity Source/LConn1 -- Mechanical Rotational Reference/LConn1 -- Rotational Hard Stop1/LConn1
  Rotational Hard Stop1/RConn1 -- Ideal Torque Sensor/RConn1
  Ideal Torque Sensor/RConn2 -- T/RConn1
  Ideal Torque Sensor/LConn1 -- Ideal Angular Velocity Source/RConn2

== system Pong3D/Robot 1/Joint5/Limit Joint 4 Y ==
  Ideal Angular Velocity Source : fl_lib/Mechanical/Mechanical Sources/Ideal Angular Velocity Source
  Ideal Torque Sensor : fl_lib/Mechanical/Mechanical Sensors/Ideal Torque Sensor
  Mechanical Rotational Reference : fl_lib/Mechanical/Rotational Elements/Mechanical Rotational Reference
  Rotational Hard Stop1 : fl_lib/Mechanical/Rotational Elements/Rotational Hard Stop  upper_bnd=Robot1.Joint.Upper_Bound(5) - Robot1.Joint.Initial_Angle(5) deg  lower_bnd=Robot1.Joint.Lower_Bound(5) - Robot1.Joint.Initial_Angle(5) deg  stiff_up=Robot1.Joint.Contact_Stiffness(5) N*m/rad  stiff_low=Robot1.Joint.Contact_Stiffness(5) N*m/rad  D_up=Robot1.Joint.Contact_Damping(5) N*m/(rad/s)  D_low=Robot1.Joint.Contact_Damping(5) N*m/(rad/s)  w_specify=off  w_priority=High  w=0 rad/s  t_specify=off  t_priority=High  t=0 N*m  phi_specify=off  phi_priority=High  phi=0 rad
  T : PMIOPort  Port=1  Side=Right
  W : PMIOPort  Port=2  Side=Left
  connections:
  Ideal Torque Sensor/LConn1 -- Ideal Angular Velocity Source/RConn2
  Ideal Torque Sensor/RConn2 -- T/RConn1
  Rotational Hard Stop1/RConn1 -- Ideal Torque Sensor/RConn1
  Rotational Hard Stop1/LConn1 -- Mechanical Rotational Reference/LConn1 -- Ideal Angular Velocity Source/LConn1
  W/RConn1 -- Ideal Angular Velocity Source/RConn1

== system Pong3D/Robot 1/Joint6/Limit Joint 4 Y ==
  Ideal Angular Velocity Source : fl_lib/Mechanical/Mechanical Sources/Ideal Angular Velocity Source
  Ideal Torque Sensor : fl_lib/Mechanical/Mechanical Sensors/Ideal Torque Sensor
  Mechanical Rotational Reference : fl_lib/Mechanical/Rotational Elements/Mechanical Rotational Reference
  Rotational Hard Stop1 : fl_lib/Mechanical/Rotational Elements/Rotational Hard Stop  upper_bnd=Robot1.Joint.Upper_Bound(6) - Robot1.Joint.Initial_Angle(6) deg  lower_bnd=Robot1.Joint.Lower_Bound(6) - Robot1.Joint.Initial_Angle(6) deg  stiff_up=Robot1.Joint.Contact_Stiffness(6) N*m/rad  stiff_low=Robot1.Joint.Contact_Stiffness(6) N*m/rad  D_up=Robot1.Joint.Contact_Damping(6) N*m/(rad/s)  D_low=Robot1.Joint.Contact_Damping(6) N*m/(rad/s)  w_specify=off  w_priority=High  w=0 rad/s  t_specify=off  t_priority=High  t=0 N*m  phi_specify=off  phi_priority=High  phi=0 rad
  T : PMIOPort  Port=1  Side=Right
  W : PMIOPort  Port=2  Side=Left
  connections:
  W/RConn1 -- Ideal Angular Velocity Source/RConn1
  Ideal Angular Velocity Source/LConn1 -- Mechanical Rotational Reference/LConn1 -- Rotational Hard Stop1/LConn1
  Rotational Hard Stop1/RConn1 -- Ideal Torque Sensor/RConn1
  Ideal Torque Sensor/RConn2 -- T/RConn1
  Ideal Torque Sensor/LConn1 -- Ideal Angular Velocity Source/RConn2

== system Pong3D/Robot 2/Joint1/Limit Joint 1 ==
  Ideal Angular Velocity Source : fl_lib/Mechanical/Mechanical Sources/Ideal Angular Velocity Source
  Ideal Torque Sensor : fl_lib/Mechanical/Mechanical Sensors/Ideal Torque Sensor
  Mechanical Rotational Reference : fl_lib/Mechanical/Rotational Elements/Mechanical Rotational Reference
  Rotational Hard Stop1 : fl_lib/Mechanical/Rotational Elements/Rotational Hard Stop  upper_bnd=Robot2.Joint.Upper_Bound(1) - Robot2.Joint.Initial_Angle(1) deg  lower_bnd=Robot2.Joint.Lower_Bound(1) - Robot2.Joint.Initial_Angle(1) deg  stiff_up=Robot2.Joint.Contact_Stiffness(1) N*m/rad  stiff_low=Robot2.Joint.Contact_Stiffness(1) N*m/rad  D_up=Robot2.Joint.Contact_Damping(1) N*m/(rad/s)  D_low=Robot2.Joint.Contact_Damping(1) N*m/(rad/s)  w_specify=off  w_priority=High  w=0 rad/s  t_specify=off  t_priority=High  t=0 N*m  phi_specify=off  phi_priority=High  phi=0 rad
  T : PMIOPort  Port=1  Side=Right
  W : PMIOPort  Port=2  Side=Left
  connections:
  Ideal Torque Sensor/LConn1 -- Ideal Angular Velocity Source/RConn2
  Ideal Torque Sensor/RConn2 -- T/RConn1
  Rotational Hard Stop1/RConn1 -- Ideal Torque Sensor/RConn1
  Rotational Hard Stop1/LConn1 -- Mechanical Rotational Reference/LConn1 -- Ideal Angular Velocity Source/LConn1
  W/RConn1 -- Ideal Angular Velocity Source/RConn1

== system Pong3D/Robot 2/Joint2/Limit Joint 2 ==
  Ideal Angular Velocity Source : fl_lib/Mechanical/Mechanical Sources/Ideal Angular Velocity Source
  Ideal Torque Sensor : fl_lib/Mechanical/Mechanical Sensors/Ideal Torque Sensor
  Mechanical Rotational Reference : fl_lib/Mechanical/Rotational Elements/Mechanical Rotational Reference
  Rotational Hard Stop1 : fl_lib/Mechanical/Rotational Elements/Rotational Hard Stop  upper_bnd=Robot2.Joint.Upper_Bound(2) - Robot2.Joint.Initial_Angle(2) deg  lower_bnd=Robot2.Joint.Lower_Bound(2) - Robot2.Joint.Initial_Angle(2) deg  stiff_up=Robot2.Joint.Contact_Stiffness(2) N*m/rad  stiff_low=Robot2.Joint.Contact_Stiffness(2) N*m/rad  D_up=Robot2.Joint.Contact_Damping(2) N*m/(rad/s)  D_low=Robot2.Joint.Contact_Damping(2) N*m/(rad/s)  w_specify=off  w_priority=High  w=0 rad/s  t_specify=off  t_priority=High  t=0 N*m  phi_specify=off  phi_priority=High  phi=0 rad
  T : PMIOPort  Port=1  Side=Right
  W : PMIOPort  Port=2  Side=Left
  connections:
  W/RConn1 -- Ideal Angular Velocity Source/RConn1
  Ideal Angular Velocity Source/LConn1 -- Mechanical Rotational Reference/LConn1 -- Rotational Hard Stop1/LConn1
  Rotational Hard Stop1/RConn1 -- Ideal Torque Sensor/RConn1
  Ideal Torque Sensor/RConn2 -- T/RConn1
  Ideal Torque Sensor/LConn1 -- Ideal Angular Velocity Source/RConn2

== system Pong3D/Robot 2/Joint3/Limit Joint 3 ==
  Ideal Angular Velocity Source : fl_lib/Mechanical/Mechanical Sources/Ideal Angular Velocity Source
  Ideal Torque Sensor : fl_lib/Mechanical/Mechanical Sensors/Ideal Torque Sensor
  Mechanical Rotational Reference : fl_lib/Mechanical/Rotational Elements/Mechanical Rotational Reference
  Rotational Hard Stop1 : fl_lib/Mechanical/Rotational Elements/Rotational Hard Stop  upper_bnd=Robot2.Joint.Upper_Bound(3) - Robot2.Joint.Initial_Angle(3) deg  lower_bnd=Robot2.Joint.Lower_Bound(3) - Robot2.Joint.Initial_Angle(3) deg  stiff_up=Robot2.Joint.Contact_Stiffness(3) N*m/rad  stiff_low=Robot2.Joint.Contact_Stiffness(3) N*m/rad  D_up=Robot2.Joint.Contact_Damping(3) N*m/(rad/s)  D_low=Robot2.Joint.Contact_Damping(3) N*m/(rad/s)  w_specify=off  w_priority=High  w=0 rad/s  t_specify=off  t_priority=High  t=0 N*m  phi_specify=off  phi_priority=High  phi=0 rad
  T : PMIOPort  Port=1  Side=Right
  W : PMIOPort  Port=2  Side=Left
  connections:
  Ideal Torque Sensor/LConn1 -- Ideal Angular Velocity Source/RConn2
  Ideal Torque Sensor/RConn2 -- T/RConn1
  Rotational Hard Stop1/RConn1 -- Ideal Torque Sensor/RConn1
  Rotational Hard Stop1/LConn1 -- Mechanical Rotational Reference/LConn1 -- Ideal Angular Velocity Source/LConn1
  W/RConn1 -- Ideal Angular Velocity Source/RConn1

== system Pong3D/Robot 2/Joint4/Limit Joint 4 Y ==
  Ideal Angular Velocity Source : fl_lib/Mechanical/Mechanical Sources/Ideal Angular Velocity Source
  Ideal Torque Sensor : fl_lib/Mechanical/Mechanical Sensors/Ideal Torque Sensor
  Mechanical Rotational Reference : fl_lib/Mechanical/Rotational Elements/Mechanical Rotational Reference
  Rotational Hard Stop1 : fl_lib/Mechanical/Rotational Elements/Rotational Hard Stop  upper_bnd=Robot2.Joint.Upper_Bound(4) - Robot2.Joint.Initial_Angle(4) deg  lower_bnd=Robot2.Joint.Lower_Bound(4) - Robot2.Joint.Initial_Angle(4) deg  stiff_up=Robot2.Joint.Contact_Stiffness(4) N*m/rad  stiff_low=Robot2.Joint.Contact_Stiffness(4) N*m/rad  D_up=Robot2.Joint.Contact_Damping(4) N*m/(rad/s)  D_low=Robot2.Joint.Contact_Damping(4) N*m/(rad/s)  w_specify=off  w_priority=High  w=0 rad/s  t_specify=off  t_priority=High  t=0 N*m  phi_specify=off  phi_priority=High  phi=0 rad
  T : PMIOPort  Port=1  Side=Right
  W : PMIOPort  Port=2  Side=Left
  connections:
  W/RConn1 -- Ideal Angular Velocity Source/RConn1
  Ideal Angular Velocity Source/LConn1 -- Mechanical Rotational Reference/LConn1 -- Rotational Hard Stop1/LConn1
  Rotational Hard Stop1/RConn1 -- Ideal Torque Sensor/RConn1
  Ideal Torque Sensor/RConn2 -- T/RConn1
  Ideal Torque Sensor/LConn1 -- Ideal Angular Velocity Source/RConn2

== system Pong3D/Robot 2/Joint5/Limit Joint 4 Y ==
  Ideal Angular Velocity Source : fl_lib/Mechanical/Mechanical Sources/Ideal Angular Velocity Source
  Ideal Torque Sensor : fl_lib/Mechanical/Mechanical Sensors/Ideal Torque Sensor
  Mechanical Rotational Reference : fl_lib/Mechanical/Rotational Elements/Mechanical Rotational Reference
  Rotational Hard Stop1 : fl_lib/Mechanical/Rotational Elements/Rotational Hard Stop  upper_bnd=Robot2.Joint.Upper_Bound(5) - Robot2.Joint.Initial_Angle(5) deg  lower_bnd=Robot2.Joint.Lower_Bound(5) - Robot2.Joint.Initial_Angle(5) deg  stiff_up=Robot2.Joint.Contact_Stiffness(5) N*m/rad  stiff_low=Robot2.Joint.Contact_Stiffness(5) N*m/rad  D_up=Robot2.Joint.Contact_Damping(5) N*m/(rad/s)  D_low=Robot2.Joint.Contact_Damping(5) N*m/(rad/s)  w_specify=off  w_priority=High  w=0 rad/s  t_specify=off  t_priority=High  t=0 N*m  phi_specify=off  phi_priority=High  phi=0 rad
  T : PMIOPort  Port=1  Side=Right
  W : PMIOPort  Port=2  Side=Left
  connections:
  Ideal Torque Sensor/LConn1 -- Ideal Angular Velocity Source/RConn2
  Ideal Torque Sensor/RConn2 -- T/RConn1
  Rotational Hard Stop1/RConn1 -- Ideal Torque Sensor/RConn1
  Rotational Hard Stop1/LConn1 -- Mechanical Rotational Reference/LConn1 -- Ideal Angular Velocity Source/LConn1
  W/RConn1 -- Ideal Angular Velocity Source/RConn1
